simulink library "Tire_MFSwift"  (R2026a)
settings: Solver=VariableStepAuto
undefined symbols (not defined in the file): Left, UNLOADED_RADIUS, Vehicle, VERTICAL_DAMPING, VERTICAL_STIFFNESS, Visual, X, Y, Z
libraries: nesl_utility x24, sm_lib x15, mfswift_simscape_library x2, Delft_Tyre_dtlib x1, TireBody_Systems x1, mfswift_library x1, Tire_Utilities x1, $bdroot x1
(part 1 of 2)
Description:
  | Component of Simscape Vehicle Templates Library
  | 
  | Copyright 2018-2026 The MathWorks, Inc.
settings Model: Creator=smiller  LastModifiedBy=smiller

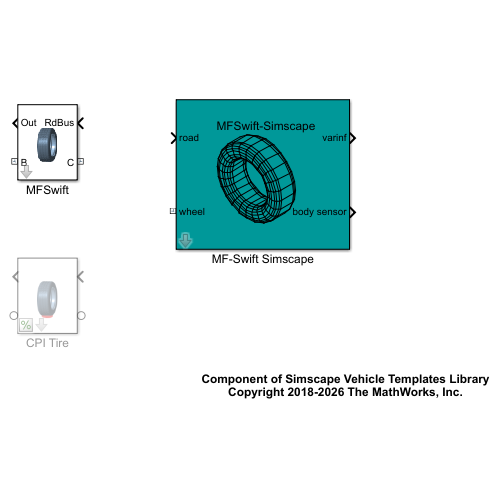
[thumbnail: Simulink's stored preview of the top-level diagram]
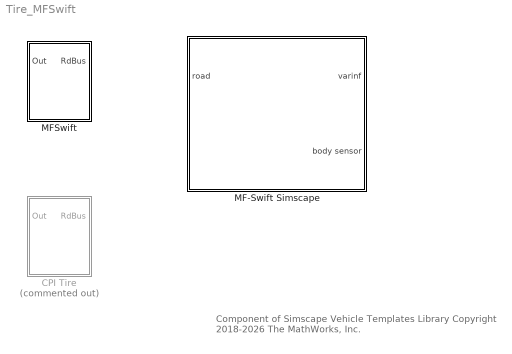
== system Tire_MFSwift ==
  note: Component of Simscape Vehicle Templates Library
      | Copyright 2018-2026 The MathWorks, Inc.
  CPI Tire : Subsystem  Commented=on  VariantControl=CPI  mask{idtyre=0}
      mask prompts: idtyre "Tyre ID [integer]"
      mask Display: image('sm_car_vehicle_tire_delftcpi_IMAGE.png');
  MF-Swift Simscape : Subsystem  Tag=STI tyre  mask(MF-Tyre/MF-Swift Simscape tire){idtyre=1, inertia=[10 1 2], tpfname=which('car213_40R21.tir'), rdfname='', road_mode=(1xxxx) default flat, side_mode=(x1xxx) left, cnt_mode=(xx1xx) smooth road, dyn_mode=(xxx2x) relaxation behaviour - non-linear, mf_mode=(xxxx4) combined, overwrite=off, use_mode=1e8, tv_model=Disabled, internal_solver=off, disp_debug=off, popup_leftRight=Left}
      mask prompts: idtyre "Tyre ID [integer]"; inertia "Rim inertia [3x real] mass(kg) Ixx Iyy (kgm2)"; tpfname "Tire properties file [string] or Tire struct [data structure]"; rdfname "Road data file [string]"; road_mode "Road method          :"; side_mode "Tyre side                :"; cnt_mode "Contact method       :"; dyn_mode "Dynamics               :"; mf_mode "Slip forces              :"; overwrite "Overwrite use mode with:"; tv_model "T&&V model               :"; internal_solver "Activate internal RK4 solver"; disp_debug "Display debug messages"; popup_leftRight "Left/Right"
      mask help:
      | MF-Tyre/MF-Swift tire model. Inputs to the tire are the motions at the wheel centre. The force and torque outputs correspond to the forces at the wheel center.
      |
      | Tire model version: MF-Tyre/MF-Swift v2021.1
      | © 2021 Siemens Industry Software and Services B.V.
      mask init:
      | curblk = gcb;
      | 
      | %radius     = 1;
      | %width      = 1;
      | %belt_mass  = 1;
      | %belt_Ixx   = 1;
      | %belt_Iyy   = 1;
      | %tyre_mass  = 1;
      | %tyre_Ixx   = 1;
      | %tyre_Iyy   = 1;
      | %mass = 1;
      | %wheelbody  = [10 1 2];
      | %Imat = [1 0 0; 0 1 0; 0 0 1];
      | 
      | idroad=1;
      | if(idtyre >= 10000 || idtyre <= 0)
      |     error('Invalid tire ID. Valid range is: 1-9999')
      | end
      | if(0 == strcmp(bdroot, 'mfswift_simscape_library'))
      |     solver_type = get_param(bdroot,'Solver');
      |     if (internal_solver)
      |         idtyre = idtyre + 10000;
      |         if(0 == strcmp(solver_type, 'ode1') && (disp_debug))
      |             warning(['ode1 solver should be used when using internal RK4 solver for more stable results'])
      |         end
      |     else
      |         if (0 == strcmp(solver_type, 'ode4')&& (disp_debug))
      |             % Disabled warning
      |             %warning(['It is recommended to use ode4 solver with external solver for more stable results'])
      |         end
      |     end
      | end
      | 
      | if strcmp(get_param(gcb,'overwrite'),'off')
      |     if cnt_mode == 3
      |         contact = 5;
      |     elseif cnt_mode == 2
      |         contact = 3;
      |     else
      |         contact = 1;
      |     end
      |     
      |     iswtch = 10000*road_mode + 1000*side_mode + 100*contact + 10*(dyn_mode-1) + (mf_mode-1);
      |     
      |     if (disp_debug) disp(['Delft-Tyre ' num2str(idtyre) ' -> use_mode=' num2str(iswtch) ]); end
      | else
      |     iswtch=use_mode;
      | end
      | 
      | currentFolder = dir;
      | hasTir = any(strcmp(tpfname, {currentFolder(~[currentFolder.isdir]).name}));
      | 
      | override_tv_mode = -1;
      | if(tv_model == 4)
      |     override_tv_mode = 3;
      | elseif(tv_model == 3)
      |     override_tv_mode = 2;
      | elseif (tv_model == 2)
      |     override_tv_mode = 1;
      | else
      |     override_tv_mode = 0;
      | end
      | 
      | typarr_updated = 0;
      | if (isstruct(tpfname))
      |     if(isfield(tpfname.MODEL, 'FITTYP'))
      |         if(tv_mode_override > 0)
      |             if(tpfname.MODEL.FITTYP < 70)
      |                 warning('For FITTYP less than 70, the T&V model is not available. The selected T&V mode will be ignored');
      |             else
      |                 tpfname.MODEL.TV_MODEL = tv_mode_override;
      |             end
      |         end
      |     end
      |     typarr = m_mfswift_struct2array(tpfname);
      |     typarr_updated = 1;
      | elseif (length(tpfname) == 0)
      |     %continue
      | elseif (hasTir == 1)
      |     typarr = m_mfswift_tirparser(tpfname, 'TV_MODE', override_tv_mode);
      |     typarr_updated = 1;
      | elseif (ischar(tpfname) && strcmp('', which(tpfname)) == 0)
      |     typarr = m_mfswift_tirparser(which(tpfname), 'TV_MODE', override_tv_mode);
      |     typarr_updated = 1;
      | else
      |     warning(['Mask parameter ''Tire property file'' should be supplied as string for tire ' num2str(idtyre)])
      |     if(length(tpfname) ~= 0)
      |         warning(['Make sure that " ' tpfname ' " is named correctly and it is available on the Matlab path or exists in the current working directory.'])
      |     end
      | end
      | 
      | tyreSimulationMode = get_param(bdroot, 'SimulationMode');
      | tyreTargetFile = get_param(bdroot, 'SystemTargetFile');
      | serialization = mfs_global_setting('serialization');
      | force_entitlement = getenv('MFSWIFTRT_FORCE_ENTITLEMENT');
      | 
      | if strcmp(force_entitlement, '1')
      |     tyreTemplateMakefile = 'force_serialization';
      | elseif strcmp(serialization, 'true')
      |     tyreTemplateMakefile = 'force_serialization';
      | else
      |     tyreTemplateMakefile = get_param(bdroot, 'TemplateMakefile');
      | end
      | 
      | % calculate the mass of the wheelbody in the MBS environment
      | %   normally           : rim + tyre
      | %   rigid ring dynamics: rim + part of tyre (and separate rigid body inside tyre model)
      | dynmod = iswtch - 100*floor(iswtch / 100);
      | dynmod = floor(dynmod / 10);
      | if (length(tpfname) == 0)
      |     %continue
      | else
      |     wheelbody = m_mfswift_wheel_property('tire_properties', tpfname, 'rim_properties', inertia, 'dynamics_mode', dynmod);
      | end
      | 
      | wheelbody_mass = wheelbody(1);
      | wheelbody_Ixx  = wheelbody(2);
      | wheelbody_Iyy  = wheelbody(3);
      | 
      | % display the use_mode of the model
      | if (disp_debug) disp(['MF-Tyre/MF-Swift ' num2str(idtyre) ' -> use_mode= ' num2str(iswtch) ]); end
      |     
      | % check and calculate inertia of the rim_body
      | %if  (inertia(1) <= 0 | inertia(2) <= 0 | inertia(3) <= 0 | wheelbody_mass <= 0 | wheelbody_Ixx <= 0 | wheelbody_Iyy <= 0 )
      | if  (wheelbody_mass <= 0 | wheelbody_Ixx <= 0 | wheelbody_Iyy <= 0 )
      |      error('Initialisation calculation results in a negative mass and/or inertia!')
      |      disp_debug=1;
      | end
      |     
      | if (disp_debug)
      |     msg=['Wheel mass = ',wheelbody_mass,' kg'];
      |     disp(msg);
      |     msg=['Wheel Ixx  = ',wheelbody_Ixx,' kgm2'];
      |     disp(msg);
      |     msg=['Wheel Iyy  = ',wheelbody_Iyy,' kgm2'];
      |     disp(msg);
      | end
      | 
      | %mass = wheelbody_mass;
      | tyre_mass = wheelbody_mass;
      | tyre_Ixx  = wheelbody_Ixx;
      | tyre_Iyy  = wheelbody_Iyy;
      | 
      | %Imat = [wheelbody_Ixx 0 0; 0 wheelbody_Iyy 0; 0 0 wheelbody_Ixx];
      | 
      | %initialize road file as uint8 with terminator character.
      | roadfile=uint8([rdfname 0]);
      | 
      | fliplr = 0;
      | % CHANGE GEOMETRY ORIENTATION IF WHEEL IS ON RIGHT SIDE
      | if (side_mode == 2)
      |     fliplr = 1;
      |     %disp(['Tyre ID = ' num2str(idtyre) ', fliplr = ' num2str(fliplr)]);
      | end
      | 
      | % Parameters needed for generic tire geometry
      | tirparams   = mfeval.readTIR(tpfname);
      | tire_radius = tirparams.UNLOADED_RADIUS;
      | tire_width  = tirparams.WIDTH;
      | rim_width   = tire_width*0.1;
      | rim_radius  = tirparams.RIM_RADIUS;
      mask Help: eval('mfs_open_help()')
      mask TypeOptions road_mode: (1xxxx) default flat | (2xxxx) opencrg | (3xxxx) external
      mask Callback road_mode:
      | enables = get_param(gcb, 'MaskEnables');
      | road = get_param(gcb,'road_mode');
      | if(road(2) == '2')
      |     enables{4} = 'on';
      | else
      |     enables{4} = 'off';
      | end
      | set_param(gcb, 'MaskEnables', enables);
      mask TypeOptions side_mode: (x1xxx) left | (x2xxx) right | (x3xxx) symmetric | (x4xxx) mirror
      mask TypeOptions cnt_mode: (xx1xx) smooth road | (xx3xx) moving road | (xx5xx) enveloping
      mask TypeOptions dyn_mode: (xxx0x) steady-state | (xxx1x) relaxation behaviour | (xxx2x) relaxation behaviour - non-linear | (xxx3x) rigid-ring
      mask TypeOptions mf_mode: (xxxx0) none | (xxxx1) longitudinal | (xxxx2) lateral | (xxxx3) uncombined | (xxxx4) combined | (xxxx5) combined+turnslip
      mask Callback overwrite:
      | enables = get_param(gcb, 'MaskEnables');
      | if strcmp(get_param(gcb,'overwrite'),'on')
      |     enables{4} = 'on';
      | 
      |     enables{5} = 'off';
      |     enables{6} = 'off';
      |     enables{7} = 'off';
      |     enables{8} = 'off';
      |     enables{9} = 'off';
      | 
      |     enables{11} = 'on';
      | else
      |     road = get_param(gcb,'road_mode');
      |     if(road(2) == '2')
      |         enables{4} = 'on';
      |     else
      |         enables{4} = 'off';
      |     end
      | 
      |     enables{5} = 'on';
      |     enables{6} = 'on';
      |     enables{7} = 'on';
      |     enables{8} = 'on';
      |     enables{9} = 'on';
      | 
      |     enables{11} = 'off';
      | end
      | set_param(gcb, 'MaskEnables', enables);
      mask TypeOptions tv_model: Disabled | Static | Dynamic without IP | Dynamic with IP
      mask TypeOptions popup_leftRight: Tire Body/popup_leftRight
      mask DialogControl cont_vis Prompt: Visualization
      mask Display:
      | text(0.3*115,0.7*178,'  MFSwift-Simscape')
      | plot(89.*[0.8828 0.8769 0.8597 0.7299 0.7043 0.6745 0.6443 0.6195 0.5884 0.5712 0.5653 0.5573 0.5346 0.4985 0.4515 0.3965 0.3373 ]+160/2-0.43*89,89.*[0.3654 0.3482 0.3335 0.2583 0.2486 0.2453 0.2486 0.2583 0.2764 0.2911 0.3083 0.2449 0.1945 0.1609 0.1462 0.1520 0.1768 ]+0.3*89)
      | plot(89.*[0.3255 0.3889 0.3965 0.4112 0.4313 0.3767 ]+160/2-0.43*89,89.*[0.1491 0.1222 0.1520 0.1777 0.1949 0.2184 ]+0.3*89)
      | plot(89.*[0.3553 0.4112 0.4633 0.4826 0.5464 ]+160/2-0.43*89,89.*[0.2012 0.1777 0.1722 0.1898 0.2268 ]+0.3*89)
      | plot(89.*[0.5426 0.5262 0.4826 0.4313 0.5603 0.5603 0.5065 ]+160/2-0.43*89,89.*[0.2184 0.2037 0.1898 0.1949 0.2692 0.2701 0.2932 ]+0.3*89)
      | plot(89.*[0.5279 0.5460 0.4868 ]+160/2-0.43*89,89.*[0.3007 0.2969 0.3402 ]+0.3*89)
      | plot(89.*[0.5279 0.5624 ]+160/2-0.43*89,89.*[0.3007 0.2856 ]+0.3*89)
      | plot(89.*[0.5628 0.5460 ]+160/2-0.43*89,89.*[0.2898 0.2969 ]+0.3*89)
      | plot(89.*[0.5712 0.5628 0.5573 ]+160/2-0.43*89,89.*[0.2911 0.2222 0.2449 ]+0.3*89)
      | plot(89.*[0.5586 0.5422 0.5082 0.4633 0.4515 0.4481 0.3889 0.3902 0.4544 0.5099 0.5523 0.5792 0.5884 ]+160/2-0.43*89,89.*[0.2541 0.2180 0.1861 0.1722 0.1462 0.1163 0.1222 0.0928 0.0865 0.1033 0.1428 0.2016 0.2764 ]+0.3*89)
      | plot(89.*[0.6195 0.6090 0.5792 0.5628 0.5380 0.5346 0.5422 ]+160/2-0.43*89,89.*[0.2583 0.1751 0.2016 0.2222 0.1680 0.1945 0.2180 ]+0.3*89)
      | plot(89.*[0.5262 0.5082 0.4985 0.4994 0.5380 0.5523 0.5792 0.6090 0.6333 0.6443 ]+160/2-0.43*89,89.*[0.2037 0.1861 0.1609 0.1319 0.1680 0.1428 0.1092 0.1751 0.1596 0.2486 ]+0.3*89)
      | plot(89.*[0.6745 0.6627 0.6333 0.6018 0.5792 0.5317 0.5099 0.4994 0.4481 0.4544 0.4700 0.5317 0.5510 0.6018 0.6291 0.6627 0.6926 0.7043 ]+160/2-0.43*89,89.*[0.2453 0.1508 0.1596 0.0890 0.1092 0.0655 0.1033 0.1319 0.1163 0.0865 0.0462 0.0655 0.0416 0.0890 0.0764 0.1508 0.1508 0.2486 ]+0.3*89)
      | plot(89.*[0.7299 0.7178 0.6926 0.6577 0.6291 0.5758 0.5510 0.4851 0.4700 0.3986 0.3213 0.2440 0.1718 0.1100 0.0626 ]+160/2-0.43*89,89.*[0.2583 0.1596 0.1508 0.0739 0.0764 0.0269 0.0416 0.0210 0.0462 0.0533 0.0861 0.1424 0.2184 0.3087 0.4074 ]+0.3*89)
      | plot(89.*[0.0487 0.0995 0.1100 0.1323 0.1516 0.1760 0.1399 ]+160/2-0.43*89,89.*[0.4082 0.3028 0.3087 0.3213 0.3326 0.3469 0.4221 ]+0.3*89)
      | plot(89.*[0.1126 0.1516 0.2024 0.2234 0.2474 0.2709 0.4011 0.4200 0.4322 0.3847 0.3486 0.3255 ]+160/2-0.43*89,89.*[0.4141 0.3326 0.2579 0.2776 0.2969 0.3121 0.3872 0.3965 0.3982 0.4670 0.5426 0.6191 ]+0.3*89)
      | plot(89.*[0.3486 0.3410 0.3755 0.3847 ]+160/2-0.43*89,89.*[0.5426 0.5330 0.4616 0.4670 ]+0.3*89)
      | plot(89.*[0.3755 0.3570 0.3234 ]+160/2-0.43*89,89.*[0.4616 0.4511 0.5212 ]+0.3*89)
      | plot(89.*[0.3570 0.2272 0.1936 ]+160/2-0.43*89,89.*[0.4511 0.3759 0.4460 ]+0.3*89)
      | plot(89.*[0.1684 0.2029 0.2272 0.2709 0.3217 0.4519 0.4721 0.4868 0.4322 ]+160/2-0.43*89,89.*[0.4334 0.3625 0.3759 0.3121 0.2583 0.3331 0.3415 0.3402 0.3982 ]+0.3*89)
      | plot(89.*[0.4200 0.3755 ]+160/2-0.43*89,89.*[0.3965 0.4616 ]+0.3*89)
      | plot(89.*[0.3570 0.4011 0.4519 0.5065 0.5279 0.4721 0.4200 ]+160/2-0.43*89,89.*[0.4511 0.3872 0.3331 0.2932 0.3007 0.3415 0.3965 ]+0.3*89)
      | plot(89.*[0.5065 0.3767 0.3217 0.2995 0.2474 0.2029 0.1760 0.2234 0.2785 0.2995 0.3553 0.3767 ]+160/2-0.43*89,89.*[0.2932 0.2184 0.2583 0.2419 0.2969 0.3625 0.3469 0.2776 0.2197 0.2419 0.2012 0.2184 ]+0.3*89)
      | plot(89.*[0.3553 0.3373 0.2785 0.2617 0.2024 0.1873 0.1323 0.0899 0.0630 0.0542 0.0231 0.0059 0.0000 0.0113 0.0168 0.0332 0.0630 0.0878 0.1172 0.1470 0.1722 0.3024 0.3192 0.3255 0.3179 0.3121 0.2948 0.1651 0.1394 0.1470 0.1172 0.0878 0.0630 0.0332 0.0168 0.0113 0.0000 ]+160/2-0.43*89,89.*[0.2012 0.1768 0.2197 0.1957 0.2579 0.2402 0.3213 0.4099 0.4994 0.5846 0.6027 0.6174 0.6346 0.5271 0.5157 0.5078 0.4994 0.4964 0.4990 0.5061 0.5174 0.5922 0.6056 0.6191 0.6917 0.6745 0.6598 0.5846 0.5745 0.6350 0.6350 0.6434 0.6594 0.6858 0.7064 0.7291 0.6346 ]+0.3*89)
      | plot(89.*[0.0059 0.0168 ]+160/2-0.43*89,89.*[0.6174 0.7064 ]+0.3*89)
      | plot(89.*[0.0113 0.0454 0.0529 0.0181 0.0113 ]+160/2-0.43*89,89.*[0.7291 0.8034 0.8270 0.7497 0.7291 ]+0.3*89)
      | plot(89.*[0.0168 0.0487 0.0454 ]+160/2-0.43*89,89.*[0.7064 0.7770 0.8034 ]+0.3*89)
      | plot(89.*[0.0487 0.0626 0.0899 0.0630 0.0542 0.0794 0.0878 0.1126 0.0899 ]+160/2-0.43*89,89.*[0.7770 0.7518 0.7182 0.6594 0.5846 0.5745 0.6434 0.6976 0.7182 ]+0.3*89)
      | plot(89.*[0.1126 0.1399 0.1684 0.1936 0.2570 ]+160/2-0.43*89,89.*[0.6976 0.6854 0.6829 0.6905 0.7274 ]+0.3*89)
      | plot(89.*[0.3011 0.1722 0.1936 ]+160/2-0.43*89,89.*[0.7182 0.6438 0.6905 ]+0.3*89)
      | plot(89.*[0.1684 0.1470 0.1722 0.1651 0.1722 0.1936 0.3234 0.3410 0.3192 0.3121 0.3163 ]+160/2-0.43*89,89.*[0.6829 0.6350 0.6438 0.5846 0.5174 0.4460 0.5212 0.5330 0.6056 0.6745 0.7119 ]+0.3*89)
      | plot(89.*[0.3200 0.3179 ]+160/2-0.43*89,89.*[0.7102 0.6917 ]+0.3*89)
      | plot(89.*[0.3020 0.2948 0.3024 0.3234 ]+160/2-0.43*89,89.*[0.7178 0.6598 0.5922 0.5212 ]+0.3*89)
      | plot(89.*[0.1470 0.1394 0.1096 0.1172 0.1399 0.1760 0.1516 0.1323 0.1100 0.0995 0.0987 0.1688 0.1806 0.1999 0.3297 0.2566 0.1264 0.0701 0.0529 0.1084 0.1264 0.1999 ]+160/2-0.43*89,89.*[0.5061 0.5745 0.5716 0.6350 0.6854 0.7190 0.7341 0.7577 0.7959 0.8240 0.8530 0.8748 0.9005 0.9185 0.9933 0.9706 0.8958 0.8438 0.8270 0.8782 0.8958 0.9185 ]+0.3*89)
      | plot(89.*[0.1806 0.1084 0.0987 0.0454 ]+160/2-0.43*89,89.*[0.9005 0.8782 0.8530 0.8034 ]+0.3*89)
      | plot(89.*[0.0487 0.0995 0.1655 0.1688 ]+160/2-0.43*89,89.*[0.7770 0.8240 0.8446 0.8748 ]+0.3*89)
      | plot(89.*[0.1655 0.1718 0.1873 0.2024 0.2234 0.2474 0.2029 0.1760 0.2234 ]+160/2-0.43*89,89.*[0.8446 0.8148 0.7745 0.7497 0.7333 0.7283 0.7144 0.7190 0.7333 ]+0.3*89)
      | plot(89.*[0.2272 0.2478 ]+160/2-0.43*89,89.*[0.7215 0.7278 ]+0.3*89)
      | plot(89.*[0.2272 0.2029 0.1684 ]+160/2-0.43*89,89.*[0.7215 0.7144 0.6829 ]+0.3*89)
      | plot(89.*[0.1936 0.2272 ]+160/2-0.43*89,89.*[0.6905 0.7215 ]+0.3*89)
      | plot(89.*[0.2024 0.1516 0.1126 ]+160/2-0.43*89,89.*[0.7497 0.7341 0.6976 ]+0.3*89)
      | plot(89.*[0.0899 0.1323 0.1873 0.2520 0.2440 0.2428 0.2499 0.2650 0.2852 0.4150 0.4372 0.3528 0.3297 0.4150 0.5065 0.5279 0.5460 0.4586 0.4372 0.5279 ]+160/2-0.43*89,89.*[0.7182 0.7577 0.7745 0.7686 0.8076 0.8370 0.8669 0.8925 0.9097 0.9849 0.9920 1.0000 0.9933 0.9849 0.9458 0.9534 0.9500 0.9870 0.9920 0.9534 ]+0.3*89)
      | plot(89.*[0.5065 0.3767 0.2852 0.1999 ]+160/2-0.43*89,89.*[0.9458 0.8711 0.9097 0.9185 ]+0.3*89)
      | plot(89.*[0.1806 0.2650 0.3553 0.3767 ]+160/2-0.43*89,89.*[0.9005 0.8925 0.8538 0.8711 ]+0.3*89)
      | plot(89.*[0.3553 0.3373 0.2499 0.1688 ]+160/2-0.43*89,89.*[0.8538 0.8295 0.8669 0.8748 ]+0.3*89)
      | plot(89.*[0.1655 0.2428 0.3255 0.3373 ]+160/2-0.43*89,89.*[0.8446 0.8370 0.8018 0.8295 ]+0.3*89)
      | plot(89.*[0.3255 0.3213 0.3213 0.3255 0.3373 0.2785 0.2617 0.3255 ]+160/2-0.43*89,89.*[0.8018 0.7749 0.7388 0.7165 0.7031 0.7278 0.7438 0.7165 ]+0.3*89)
      | plot(89.*[0.3213 0.2520 0.2617 0.2024 ]+160/2-0.43*89,89.*[0.7388 0.7686 0.7438 0.7497 ]+0.3*89)
      | plot(89.*[0.2234 0.2785 ]+160/2-0.43*89,89.*[0.7333 0.7278 ]+0.3*89)
      | plot(89.*[0.2869 0.2474 ]+160/2-0.43*89,89.*[0.7241 0.7283 ]+0.3*89)
      | plot(89.*[0.2440 0.3213 0.3986 0.4078 0.4246 0.4456 0.4683 0.5981 0.6182 0.6329 0.5460 ]+160/2-0.43*89,89.*[0.8076 0.7749 0.7186 0.7417 0.7661 0.7879 0.8043 0.8790 0.8874 0.8862 0.9500 ]+0.3*89)
      | plot(89.*[0.5279 0.6182 0.7022 0.7140 0.6329 ]+160/2-0.43*89,89.*[0.9534 0.8874 0.7984 0.8001 0.8862 ]+0.3*89)
      | plot(89.*[0.5981 0.5065 ]+160/2-0.43*89,89.*[0.8790 0.9458 ]+0.3*89)
      | plot(89.*[0.5981 0.6829 0.7022 ]+160/2-0.43*89,89.*[0.8790 0.7892 0.7984 ]+0.3*89)
      | plot(89.*[0.6829 0.5535 0.4683 0.3767 ]+160/2-0.43*89,89.*[0.7892 0.7144 0.8043 0.8711 ]+0.3*89)
      | plot(89.*[0.3553 0.4456 0.5300 0.5535 ]+160/2-0.43*89,89.*[0.8538 0.7879 0.6989 0.7144 ]+0.3*89)
      | plot(89.*[0.5300 0.5061 0.4246 0.3373 ]+160/2-0.43*89,89.*[0.6989 0.6800 0.7661 0.8295 ]+0.3*89)
      | plot(89.*[0.3255 0.4078 0.4851 0.5061 ]+160/2-0.43*89,89.*[0.8018 0.7417 0.6602 0.6800 ]+0.3*89)
      | plot(89.*[0.4851 0.4700 0.3986 0.3902 0.3889 0.4481 0.4544 0.4700 ]+160/2-0.43*89,89.*[0.6602 0.6426 0.7186 0.6884 0.6703 0.6077 0.6203 0.6426 ]+0.3*89)
      | plot(89.*[0.4851 0.5510 0.5758 0.6027 0.6262 0.7560 0.7745 0.7841 0.7140 ]+160/2-0.43*89,89.*[0.6602 0.5632 0.5779 0.5930 0.6069 0.6816 0.6926 0.6980 0.8001 ]+0.3*89)
      | plot(89.*[0.7022 0.7745 ]+160/2-0.43*89,89.*[0.7984 0.6926 ]+0.3*89)
      | plot(89.*[0.7841 0.8375 0.8303 0.7745 ]+160/2-0.43*89,89.*[0.6980 0.5863 0.5766 0.6926 ]+0.3*89)
      | plot(89.*[0.7560 0.6829 ]+160/2-0.43*89,89.*[0.6816 0.7892 ]+0.3*89)
      | plot(89.*[0.7560 0.8123 0.8303 ]+160/2-0.43*89,89.*[0.6816 0.5649 0.5766 ]+0.3*89)
      | plot(89.*[0.8123 0.6825 0.6262 0.5535 ]+160/2-0.43*89,89.*[0.5649 0.4901 0.6069 0.7144 ]+0.3*89)
      | plot(89.*[0.5300 0.6027 0.6577 0.6825 ]+160/2-0.43*89,89.*[0.6989 0.5930 0.4775 0.4901 ]+0.3*89)
      | plot(89.*[0.6577 0.6291 0.5758 0.5061 ]+160/2-0.43*89,89.*[0.4775 0.4658 0.5779 0.6800 ]+0.3*89)
      | plot(89.*[0.4700 0.5317 0.5510 0.6018 0.6291 ]+160/2-0.43*89,89.*[0.6426 0.5523 0.5632 0.4578 0.4658 ]+0.3*89)
      | plot(89.*[0.6018 0.5792 0.5317 0.5099 0.4544 0.3902 0.3213 ]+160/2-0.43*89,89.*[0.4578 0.4536 0.5523 0.5397 0.6203 0.6884 0.7388 ]+0.3*89)
      | plot(89.*[0.3255 0.3889 0.3965 0.4515 0.4481 0.4994 0.5099 0.5523 0.5792 ]+160/2-0.43*89,89.*[0.7165 0.6703 0.6602 0.6018 0.6077 0.5334 0.5397 0.4511 0.4536 ]+0.3*89)
      | plot(89.*[0.6018 0.6333 0.6627 0.6926 0.7178 0.8475 0.8652 0.8711 0.8375 ]+160/2-0.43*89,89.*[0.4578 0.3503 0.3524 0.3599 0.3713 0.4460 0.4595 0.4729 0.5863 ]+0.3*89)
      | plot(89.*[0.8303 0.8652 ]+160/2-0.43*89,89.*[0.5766 0.4595 ]+0.3*89)
      | plot(89.*[0.8711 0.8828 0.8711 0.8652 0.8475 0.7178 0.6825 0.6577 0.6027 0.5758 0.5061 0.4851 0.4078 0.3986 0.3902 0.3213 0.2520 0.1873 0.1718 0.1655 0.0995 0.0987 0.1688 0.1655 0.2428 0.2440 0.2520 0.2617 0.3255 0.3373 ]+160/2-0.43*89,89.*[0.4729 0.3654 0.2713 0.2503 0.2348 0.1596 0.0815 0.0739 0.0223 0.0269 0.0050 0.0210 0.0290 0.0533 0.0928 0.1222 0.1726 0.2402 0.2184 0.2058 0.3028 0.3020 0.1999 0.2058 0.1243 0.1424 0.1726 0.1957 0.1491 0.1768 ]+0.3*89)
      | plot(89.*[0.3255 0.3213 0.3213 0.3255 0.4078 0.4246 0.5061 0.5300 0.6027 0.6262 0.6825 0.8123 0.8475 0.8597 0.8475 0.8123 ]+160/2-0.43*89,89.*[0.1491 0.1222 0.0861 0.0643 0.0290 0.0130 0.0050 0.0000 0.0223 0.0294 0.0815 0.1562 0.2348 0.3335 0.4460 0.5649 ]+0.3*89)
      | plot(89.*[0.8652 0.8769 0.8652 0.8303 0.8123 0.7560 0.6262 0.5535 0.5300 0.4456 0.4246 0.3373 0.3255 0.2428 0.2499 0.3373 ]+160/2-0.43*89,89.*[0.4595 0.3482 0.2503 0.1735 0.1562 0.1046 0.0294 0.0067 0.0000 0.0084 0.0130 0.0504 0.0643 0.1243 0.1138 0.0504 ]+0.3*89)
      | plot(89.*[0.0487 0.0168 0.0059 ]+160/2-0.43*89,89.*[0.4082 0.5157 0.6174 ]+0.3*89)
      | plot(89.*[0.0231 0.0332 0.0626 0.1100 0.1718 0.2440 ]+160/2-0.43*89,89.*[0.6027 0.6858 0.7518 0.7959 0.8148 0.8076 ]+0.3*89)
      | plot(89.*[0.3373 0.3965 ]+160/2-0.43*89,89.*[0.7031 0.6602 ]+0.3*89)
      | plot(89.*[0.4515 0.4985 0.4994 0.5380 0.5523 0.5792 0.6090 0.6333 0.6443 ]+160/2-0.43*89,89.*[0.6018 0.5330 0.5334 0.4519 0.4511 0.3612 0.3532 0.3503 0.2486 ]+0.3*89)
      | plot(89.*[0.6745 0.6627 0.6291 ]+160/2-0.43*89,89.*[0.2453 0.3524 0.4658 ]+0.3*89)
      | plot(89.*[0.6577 0.6926 0.7043 ]+160/2-0.43*89,89.*[0.4775 0.3599 0.2486 ]+0.3*89)
      | plot(89.*[0.7299 0.7178 0.6825 ]+160/2-0.43*89,89.*[0.2583 0.3713 0.4901 ]+0.3*89)
      | plot(89.*[0.5792 0.6090 0.6195 ]+160/2-0.43*89,89.*[0.4536 0.3532 0.2583 ]+0.3*89)
      | plot(89.*[0.5884 0.5792 0.5628 0.5380 0.5346 0.5573 0.5628 0.5712 ]+160/2-0.43*89,89.*[0.2764 0.3612 0.3692 0.4519 0.4578 0.3809 0.3692 0.2911 ]+0.3*89)
      | plot(89.*[0.5653 0.5573 ]+160/2-0.43*89,89.*[0.3083 0.3809 ]+0.3*89)
      | plot(89.*[0.5346 0.4985 ]+160/2-0.43*89,89.*[0.4578 0.5330 ]+0.3*89)
      | plot(89.*[0.1470 0.1684 0.1936 ]+160/2-0.43*89,89.*[0.5061 0.4334 0.4460 ]+0.3*89)
      | plot(89.*[0.1684 0.1399 0.1172 0.1096 0.0794 0.0878 0.1126 0.1399 ]+160/2-0.43*89,89.*[0.4334 0.4221 0.4990 0.5716 0.5745 0.4964 0.4141 0.4221 ]+0.3*89)
      | plot(89.*[0.1126 0.0899 0.0626 0.0332 0.0231 ]+160/2-0.43*89,89.*[0.4141 0.4099 0.4074 0.5078 0.6027 ]+0.3*89)
      | plot(89.*[0.0113 0.0454 0.0487 0.0626 ]+160/2-0.43*89,89.*[0.5271 0.4137 0.4082 0.4074 ]+0.3*89)
      | plot(89.*[0.0454 0.0987 ]+160/2-0.43*89,89.*[0.4137 0.3020 ]+0.3*89)
  MFSwift : Subsystem  VariantControl=Delft  mask(MF-Swift Tire){idtyre=2, rim_inertia=Vehicle.Chassis.TireA1.mjRim.Value, tir_name=Vehicle.Chassis.TireA1.tirFile.Value, rdf_name=Vehicle.Chassis.TireA1.roadFile.Value, tire_side_mode=(x2xxx) right, tire_contact=Vehicle.Chassis.TireA1.Contact.Value, tire_dynamics=Vehicle.Chassis.TireA1.Dynamics.Value, tire_slip=Vehicle.Chassis.TireA1.Slip.Value, solver_enable=Vehicle.Chassis.TireA1.InternalSolver.Value, TireBody=Vehicle.Chassis.TireA1.TireBody, popup_leftRight=Right, clr_tyre=Visual.Tire.clr, opc_tyre=Visual.Tire.opc, clr_rim=Visual.Rim.clr, opc_rim=Visual.Rim.opc}
      mask prompts: idtyre "Tyre ID [integer]"; rim_inertia "Rim: [Mass (kg) Ixx Iyy (kg*m2)]"; tir_name "Tyre properties [string or struct]"; rdf_name "Road data file [string]"; tire_side_mode "Tyre Side"; tire_contact "Contact Method"; tire_dynamics "Dynamics Mode"; tire_slip "Slip Mode"; solver_enable "Enable Internal Solver"; TireBody "Tire Body (structure)"; popup_leftRight "Left/Right"
      mask init:
      | curblk = gcb;
      | 
      | set_param([gcb '/Wheel and Tyre'],'cnt_mode',tire_contact);
      | set_param([gcb '/Wheel and Tyre'],'dyn_mode',tire_dynamics);
      | set_param([gcb '/Wheel and Tyre'],'mf_mode',tire_slip);
      | set_param([gcb '/Wheel and Tyre'],'tpfname',tir_name);
      | set_param([gcb '/Wheel and Tyre'],'rdfname',rdf_name);
      | 
      | % Set road_mode parameter based on road file type
      | if(contains(lower(rdf_name),'.crg'))
      |     set_param([gcb,'/Wheel and Tyre'],'road_mode','(2xxxx) opencrg');
      |     set_param([gcb,'/Road Inputs'],'LabelModeActiveChoice','NonMoving');
      | else
      |     set_param([gcb '/Wheel and Tyre'],'rdfname','''''');
      |     if(contains(lower(rdf_name),'external'))
      |         set_param([gcb,'/Wheel and Tyre'],'road_mode','(3xxxx) external');
      |         set_param([gcb,'/Road Inputs'],'LabelModeActiveChoice','ExternalRoad');
      |     else
      |         set_param([gcb,'/Wheel and Tyre'],'road_mode','(1xxxx) default flat');
      |         set_param([gcb,'/Road Inputs'],'LabelModeActiveChoice','NonMoving');
      |     end
      | end
      | 
      | % Enable or disable internal solver
      | if(strcmp(lower(solver_enable),'on'))
      |     set_param([gcb '/Wheel and Tyre'],'internal_solver','on');
      | else
      |     set_param([gcb '/Wheel and Tyre'],'internal_solver','off');
      | end
      |    
      | if(popup_leftRight == 1)
      |     set_param([gcb '/Wheel and Tyre'],'popup_leftRight','Left');
      | elseif(popup_leftRight == 2)
      |     set_param([gcb '/Wheel and Tyre'],'popup_leftRight','Right');
      | end
      mask TypeOptions idtyre: Wheel and Tyre/idtyre
      mask TypeOptions rim_inertia: Wheel and Tyre/inertia
      mask TypeOptions tire_side_mode: Wheel and Tyre/side_mode
      mask TypeOptions popup_leftRight: Left | Right
      mask TypeOptions clr_tyre: Wheel and Tyre/clr_tyre
      mask TypeOptions opc_tyre: Wheel and Tyre/opc_tyre
      mask TypeOptions clr_rim: Wheel and Tyre/clr_rim
      mask TypeOptions opc_rim: Wheel and Tyre/opc_rim
      mask DialogControl cont_tire_delft Prompt: Tire
      mask DialogControl cont_vis Prompt: Visualization
      mask DialogControl text_tire_clr Prompt: Color [RGB]
      mask DialogControl text_tire_opc Prompt: Opacity (0-1)
      mask DialogControl text_tire Prompt: Tyre
      mask DialogControl text_rim Prompt: Rim
      mask Display: image('sm_car_vehicle_tire_delft_IMAGE.png');

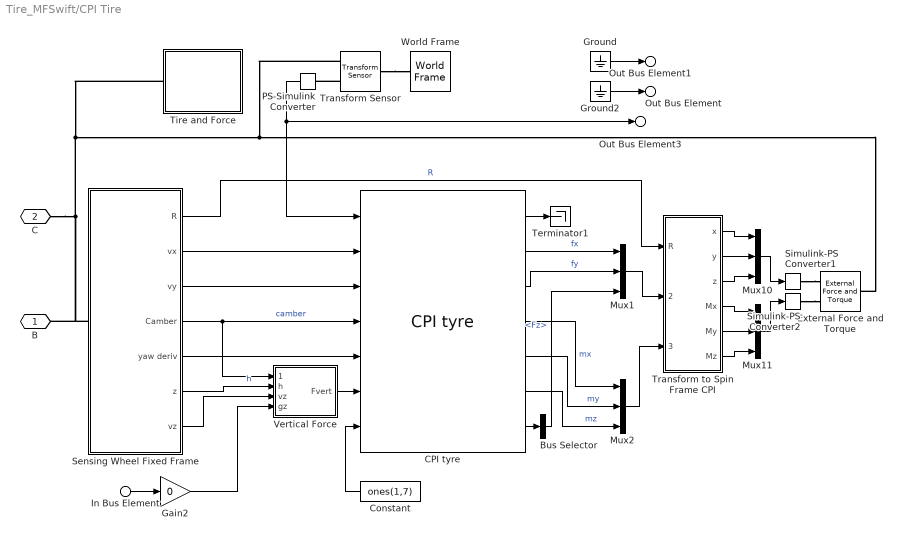
== system Tire_MFSwift/CPI Tire ==
  In Bus Element : Inport  PortName=RdBus  Element=RdBus
  Bus Selector : BusSelector  OutputSignals=Fz
  CPI tyre : Delft_Tyre_dtlib/Simulink/CPI tyre  Tag=CPI tyre  idtyre=1  tpfname=[]  side_mode=(1xxx) left  dyn_mode=(xx0x) steady-state  mf_mode=(xxx0) none  use_mode=1e8  disp_debug=off
  Constant : Constant  Value=ones(1,7)
  External Force and Torque : sm_lib/Forces and Torques/External Force and Torque  EnableForceX=off  EnableForceY=off  EnableForceZ=off  EnableForce=on  ForceResolutionFrame=AttachedFrame  EnableTorqueX=off  EnableTorqueY=off  EnableTorqueZ=off  EnableTorque=on  TorqueResolutionFrame=AttachedFrame
  Gain2 : Gain  Gain=0
  Ground : Ground
  Ground2 : Ground
  Mux{1..2,10..11} (4 alike) : Mux  Inputs=3
  PS-Simulink Converter : nesl_utility/PS-Simulink Converter  PhysicalDomain=network_engine_domain  SubClassName=ps_output  LeftPortType=input  RightPortType=output  PseudoPeriodic=off  Frequencies=[]  VectorFormat=1-D array  Unit=1  AffineConversion=off
  Sensing Wheel Fixed Frame : Subsystem
  Simulink-PS Converter1 : nesl_utility/Simulink-PS Converter  PhysicalDomain=network_engine_domain  SubClassName=ps_input  LeftPortType=input  RightPortType=output  PseudoPeriodic=off  Frequencies=[]  NoiseDistribution=none  NoiseParameters=[]  Unit=N  AffineConversion=off  FilteringAndDerivatives=provide  SimscapeFilterOrder=1  InputFilterTimeConstant=0.001  UdotUserProvided=0
  Simulink-PS Converter2 : nesl_utility/Simulink-PS Converter  PhysicalDomain=network_engine_domain  SubClassName=ps_input  LeftPortType=input  RightPortType=output  PseudoPeriodic=off  Frequencies=[]  NoiseDistribution=none  NoiseParameters=[]  Unit=N*m  AffineConversion=off  FilteringAndDerivatives=provide  SimscapeFilterOrder=1  InputFilterTimeConstant=0.001  UdotUserProvided=0
  Terminator1 : Terminator
  Tire and Force : Subsystem  mask{radius=0.4225, rim_radius=0.3048, width=0.235, rim_width=0.235*0.1, mass=10, rim_mass=0, tire_inertia=[1 2], rim_inertia=[0 0], clr_tyre_cfl=[0.5 0.5 0.5], opc_tyre_cfl=1.0, clr_rim_cfl=[0.8 0.8 0.8], opc_rim_cfl=0.5}
      mask init:
      | Imat = [tire_inertia(1)+rim_inertia(1) 0 0; 0 tire_inertia(2)+rim_inertia(2) 0; 0 0 tire_inertia(1)+rim_inertia(1)];
      mask TypeOptions clr_tyre_cfl: Tire/GraphicDiffuseColor
      mask TypeOptions opc_tyre_cfl: Tire/GraphicOpacity
      mask TypeOptions clr_rim_cfl: Rim/GraphicDiffuseColor
      mask TypeOptions opc_rim_cfl: Rim/GraphicOpacity
      mask DialogControl cont_tyre_cfl Prompt: Contact Force Tyre
      mask DialogControl group_tyre_dim Prompt: Dimensions
      mask DialogControl text_tyre_tire Prompt: Tyre
      mask DialogControl text_tyre_rim Prompt: Rim
      mask DialogControl text_tyre_dim_radius Prompt: Radius (m)
      mask DialogControl text_tyre_dim_width Prompt: Width (m)
      mask DialogControl text_tyre_mass Prompt: Mass (kg)
      mask DialogControl text_tyre_inertia Prompt: Inertia [Ixx Iyy]
      mask DialogControl cont_tyre_cfl_vis Prompt: Visualization
      mask DialogControl text_vis_tyre_cfl_clr Prompt: Color [RGB]
      mask DialogControl text_vis_tyre_cfl_opc Prompt: Opacity (0-1)
      mask DialogControl text_vis_tyre_tyre Prompt: Tyre
      mask DialogControl text_vis_tyre_rim Prompt: Rim
  Transform Sensor : sm_lib/Frames and Transforms/Transform Sensor  MeasurementFrame=NonRotatingFollower  RotationSequence=XYX  SenseAngle=off  SenseAxis=off  SenseQ=off  SenseR=off  SenseRotationSequence=off  SenseOmegaX=off  SenseOmegaY=off  SenseOmegaZ=on  SenseOmega=off  SenseQDot=off  SenseRDot=off  SenseRotationSequenceDot=off  SenseAlphaX=off  SenseAlphaY=off  SenseAlphaZ=off  SenseAlpha=off  SenseQDDot=off  SenseRDDot=off  SenseX=off  SenseY=off  SenseZ=off  SenseXYZ=off  SenseRad=off  SenseAzim=off  SenseDist=off  SenseInc=off  SenseXDot=off  SenseYDot=off  SenseZDot=off  SenseXYZDot=off  SenseRadDot=off  SenseAzimDot=off  SenseDistDot=off  SenseIncDot=off  SenseXDDot=off  SenseYDDot=off  SenseZDDot=off  SenseXYZDDot=off  SenseRadDDot=off  SenseAzimDDot=off  SenseDistDDot=off  SenseIncDDot=off
  Transform to Spin Frame CPI : Subsystem
  Vertical Force : Subsystem
  World Frame : sm_lib/Frames and Transforms/World Frame
  B : PMIOPort  Side=Right
  C : PMIOPort  Port=2  Side=Left
  Out Bus Element : Outport  VectorParamsAs1DForOutWhenUnconnected=off  PortName=Out  Element=qxyz
  Out Bus Element1 : Outport  VectorParamsAs1DForOutWhenUnconnected=off  PortName=Out  Element=xyz
  Out Bus Element3 : Outport  VectorParamsAs1DForOutWhenUnconnected=off  PortName=Out  Element=omega
  wires:
  Mux1/1 -> Transform to Spin Frame CPI/2(Fcontact)
  Mux2/1 -> Transform to Spin Frame CPI/3(MContact)
  Mux10/1 -> Simulink-PS Converter1/1
  Transform to Spin Frame CPI/2(y) -> Mux10/2
  Transform to Spin Frame CPI/3(z) -> Mux10/3
  Transform to Spin Frame CPI/5(My) -> Mux11/2
  Transform to Spin Frame CPI/4(Mx) -> Mux11/1
  Transform to Spin Frame CPI/6(Mz) -> Mux11/3
  Transform to Spin Frame CPI/1(x) -> Mux10/1
  Mux11/1 -> Simulink-PS Converter2/1
  Gain2/1 -> Vertical Force/4(gz)
  Sensing Wheel Fixed Frame/7(vz) -> Vertical Force/3(vz)
  Sensing Wheel Fixed Frame/6(z) -> Vertical Force/2(h)  "h"
  Sensing Wheel Fixed Frame/4(Camber) -> Vertical Force/1(camber), CPI tyre/4  "camber"
  CPI tyre/1 -> Terminator1/1
  PS-Simulink Converter/1 -> Out Bus Element3/1, CPI tyre/1
  Sensing Wheel Fixed Frame/2(vx) -> CPI tyre/2
  CPI tyre/4 -> Mux2/1  "mx"
  CPI tyre/3 -> Mux1/2  "fy"
  Constant/1 -> CPI tyre/7
  CPI tyre/5 -> Mux2/2  "my"
  CPI tyre/6 -> Mux2/3  "mz"
  Bus Selector/1 -> Mux1/3  "<Fz>"
  CPI tyre/2 -> Mux1/1  "fx"
  Vertical Force/1(Fvert) -> CPI tyre/6
  Sensing Wheel Fixed Frame/3(vy) -> CPI tyre/3
  Sensing Wheel Fixed Frame/5(yaw deriv) -> CPI tyre/5
  Sensing Wheel Fixed Frame/1(R) -> Transform to Spin Frame CPI/1(R)  "R"
  CPI tyre/7 -> Bus Selector/1
  Ground2/1 -> Out Bus Element/1
  Ground/1 -> Out Bus Element1/1
  In Bus Element/1 -> Gain2/1
  connections:
  Simulink-PS Converter1/RConn1 -- External Force and Torque/LConn1
  Simulink-PS Converter2/RConn1 -- External Force and Torque/LConn2
  Tire and Force/LConn1 -- Sensing Wheel Fixed Frame/LConn1 -- B/RConn1 -- C/RConn1 -- Transform Sensor/RConn1 -- External Force and Torque/RConn1
  Transform Sensor/LConn1 -- World Frame/RConn1
  Transform Sensor/RConn2 -- PS-Simulink Converter/LConn1

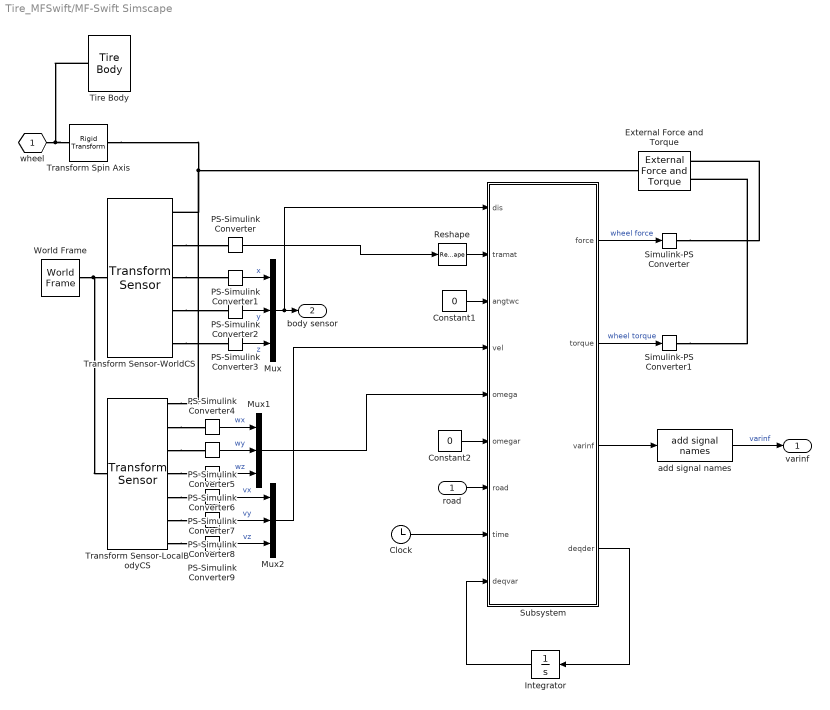
== system Tire_MFSwift/MF-Swift Simscape ==
  road : Inport
  Clock : Clock
  Constant1 : Constant  Value=0
  Constant2 : Constant  Value=0
  External Force and Torque : sm_lib/Forces and Torques/External Force and Torque  EnableForceX=off  EnableForceY=off  EnableForceZ=off  EnableForce=on  ForceResolutionFrame=AttachedFrame  EnableTorqueX=off  EnableTorqueY=off  EnableTorqueZ=off  EnableTorque=on  TorqueResolutionFrame=AttachedFrame
  Integrator : Integrator
  Mux : Mux  Inputs=3
  Mux1 : Mux  Inputs=3
  Mux2 : Mux  Inputs=3
  PS-Simulink Converter{,1..9} (10 alike) : nesl_utility/PS-Simulink Converter  PhysicalDomain=network_engine_domain  SubClassName=ps_output  LeftPortType=input  RightPortType=output  PseudoPeriodic=off  Frequencies=[]  VectorFormat=1-D array  Unit=1  AffineConversion=off
  Reshape : Reshape
  Simulink-PS Converter : nesl_utility/Simulink-PS Converter  PhysicalDomain=network_engine_domain  SubClassName=ps_input  LeftPortType=input  RightPortType=output  PseudoPeriodic=off  Frequencies=[]  NoiseDistribution=none  NoiseParameters=[]  Unit=1  AffineConversion=off  FilteringAndDerivatives=zero  SimscapeFilterOrder=1  InputFilterTimeConstant=0.001  UdotUserProvided=1
  Simulink-PS Converter1 : nesl_utility/Simulink-PS Converter  PhysicalDomain=network_engine_domain  SubClassName=ps_input  LeftPortType=input  RightPortType=output  PseudoPeriodic=off  Frequencies=[]  NoiseDistribution=none  NoiseParameters=[]  Unit=1  AffineConversion=off  FilteringAndDerivatives=zero  SimscapeFilterOrder=1  InputFilterTimeConstant=0.001  UdotUserProvided=1
  Subsystem : Subsystem
  Tire Body : TireBody_Systems/Tire Body  LabelModeActiveChoice=CAD_213_40R21  popup_leftRight=Left  TireBody=Tire.TireBody  VariantLabel=Tire.TireBody.class.Value
      settings: AttributesFormatString=%<LabelModeActiveChoice>
  Transform Sensor-LocalBodyCS : sm_lib/Frames and Transforms/Transform Sensor  MeasurementFrame=NonRotatingFollower  RotationSequence=XYX  SenseAngle=off  SenseAxis=off  SenseQ=off  SenseR=off  SenseRotationSequence=off  SenseOmegaX=on  SenseOmegaY=on  SenseOmegaZ=on  SenseOmega=off  SenseQDot=off  SenseRDot=off  SenseRotationSequenceDot=off  SenseAlphaX=off  SenseAlphaY=off  SenseAlphaZ=off  SenseAlpha=off  SenseQDDot=off  SenseRDDot=off  SenseX=off  SenseY=off  SenseZ=off  SenseXYZ=off  SenseRad=off  SenseAzim=off  SenseDist=off  SenseInc=off  SenseXDot=on  SenseYDot=on  SenseZDot=on  SenseXYZDot=off  SenseRadDot=off  SenseAzimDot=off  SenseDistDot=off  SenseIncDot=off  SenseXDDot=off  SenseYDDot=off  SenseZDDot=off  SenseXYZDDot=off  SenseRadDDot=off  SenseAzimDDot=off  SenseDistDDot=off  SenseIncDDot=off
  Transform Sensor-WorldCS : sm_lib/Frames and Transforms/Transform Sensor  MeasurementFrame=World  RotationSequence=XYX  SenseAngle=off  SenseAxis=off  SenseQ=off  SenseR=on  SenseRotationSequence=off  SenseOmegaX=off  SenseOmegaY=off  SenseOmegaZ=off  SenseOmega=off  SenseQDot=off  SenseRDot=off  SenseRotationSequenceDot=off  SenseAlphaX=off  SenseAlphaY=off  SenseAlphaZ=off  SenseAlpha=off  SenseQDDot=off  SenseRDDot=off  SenseX=on  SenseY=on  SenseZ=on  SenseXYZ=off  SenseRad=off  SenseAzim=off  SenseDist=off  SenseInc=off  SenseXDot=off  SenseYDot=off  SenseZDot=off  SenseXYZDot=off  SenseRadDot=off  SenseAzimDot=off  SenseDistDot=off  SenseIncDot=off  SenseXDDot=off  SenseYDDot=off  SenseZDDot=off  SenseXYZDDot=off  SenseRadDDot=off  SenseAzimDDot=off  SenseDistDDot=off  SenseIncDDot=off
  Transform Spin Axis : sm_lib/Frames and Transforms/Rigid Transform  RotationMethod=StandardAxis  FollAlignAxisA=+X  BaseAlignAxisA=+Y  FollAlignAxisB=+Y  BaseAlignAxisB=+Z  RotationStandardAxis=-X  RotationAngle=90  RotationAngleUnits=deg  RotationArbitraryAxis=[0 0 1]  RotationSequenceAxes=FollowerAxes  RotationSequence=XYX  RotationSequenceAngles=[0 0 0]  RotationSequenceAnglesUnits=deg  RotationMatrix=[1 0 0; 0 1 0; 0 0 1]  Quaternion=[1 0 0 0]  TranslationMethod=None  TranslationCartesianOffset=[0 0 0]  TranslationCartesianOffsetUnits=m  TranslationStandardAxis=+Z  TranslationStandardOffset=0  TranslationStandardOffsetUnits=m  TranslationROffset=0  TranslationROffsetUnits=m  TranslationThetaOffset=0  TranslationThetaOffsetUnits=deg  TranslationZOffset=0  TranslationZOffsetUnits=m
  World Frame : sm_lib/Frames and Transforms/World Frame
  add signal names : mfswift_library/MF-Swift/add signal names  SystemSampleTime=-1  VariantActivationTime=update diagram  EmptyChoice=off  PassThrough=off  PassThroughVariantControl=(default)  EmptyChoiceVariantControl=(default)  AllowFlexibleInterface=on  Latency=0  AutoFrameSizeCalculation=off
      settings: SourceProductName=MF-Tyre/MF-Swift Library
  wheel : PMIOPort  Side=Left
  varinf : Outport
  body sensor : Outport  Port=2
  wires:
  Clock/1 -> Subsystem/8(time)
  Integrator/1 -> Subsystem/9(deqvar)
  Subsystem/4(deqder) -> Integrator/1
  Subsystem/3(varinf) -> add signal names/1
  add signal names/1 -> varinf/1  "varinf"
  PS-Simulink Converter4/1 -> Mux1/1  "wx"
  PS-Simulink Converter9/1 -> Mux2/3  "vz"
  PS-Simulink Converter8/1 -> Mux2/2  "vy"
  PS-Simulink Converter7/1 -> Mux2/1  "vx"
  PS-Simulink Converter5/1 -> Mux1/2  "wy"
  Mux/1 -> Subsystem/1(dis), body sensor/1
  PS-Simulink Converter3/1 -> Mux/3  "z"
  PS-Simulink Converter2/1 -> Mux/2  "y"
  Mux2/1 -> Subsystem/4(vel)
  PS-Simulink Converter1/1 -> Mux/1  "x"
  PS-Simulink Converter6/1 -> Mux1/3  "wz"
  Mux1/1 -> Subsystem/5(omega)
  Subsystem/2(torque) -> Simulink-PS Converter1/1  "wheel torque"
  Subsystem/1(force) -> Simulink-PS Converter/1  "wheel force"
  Reshape/1 -> Subsystem/2(tramat)
  PS-Simulink Converter/1 -> Reshape/1
  Constant1/1 -> Subsystem/3(angtwc)
  road/1 -> Subsystem/7(road)
  Constant2/1 -> Subsystem/6(omegar)
  connections:
  World Frame/RConn1 -- Transform Sensor-WorldCS/LConn1 -- Transform Sensor-LocalBodyCS/LConn1
  Transform Spin Axis/LConn1 -- External Force and Torque/RConn1 -- Transform Sensor-LocalBodyCS/RConn1 -- Transform Sensor-WorldCS/RConn1
  Transform Sensor-LocalBodyCS/RConn7 -- PS-Simulink Converter9/LConn1
  Transform Sensor-WorldCS/RConn2 -- PS-Simulink Converter/LConn1
  Transform Sensor-LocalBodyCS/RConn6 -- PS-Simulink Converter8/LConn1
  Transform Sensor-WorldCS/RConn4 -- PS-Simulink Converter2/LConn1
  Transform Sensor-WorldCS/RConn3 -- PS-Simulink Converter1/LConn1
  Transform Sensor-LocalBodyCS/RConn5 -- PS-Simulink Converter7/LConn1
  Transform Sensor-WorldCS/RConn5 -- PS-Simulink Converter3/LConn1
  Transform Sensor-LocalBodyCS/RConn3 -- PS-Simulink Converter5/LConn1
  wheel/RConn1 -- Tire Body/LConn1 -- Transform Spin Axis/RConn1
  Transform Sensor-LocalBodyCS/RConn2 -- PS-Simulink Converter4/LConn1
  Transform Sensor-LocalBodyCS/RConn4 -- PS-Simulink Converter6/LConn1
  Simulink-PS Converter/RConn1 -- External Force and Torque/LConn1
  Simulink-PS Converter1/RConn1 -- External Force and Torque/LConn2

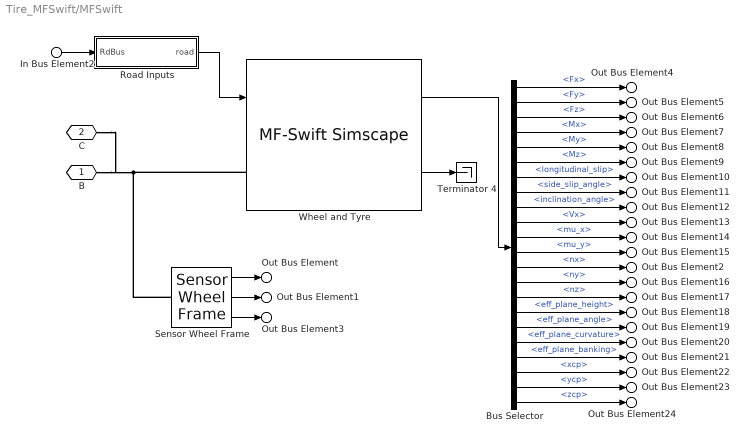
== system Tire_MFSwift/MFSwift ==
  In Bus Element2 : Inport  PortName=RdBus
  Bus Selector : BusSelector  OutputSignals=Fx,Fy,Fz,Mx,My,Mz,longitudinal_slip,side_slip_angle,inclination_angle,Vx,mu_x,mu_y,nx,ny,nz,eff_plane_height,eff_plane_angle,eff_plane_curvature,eff_plane_banking,xcp,ycp,zcp
  Road Inputs : Subsystem  Variant=on  VariantControlMode=label  LabelModeActiveChoice=ExternalRoad
  Sensor Wheel Frame : Tire_Utilities/Sensor Wheel Frame  SystemSampleTime=-1  VariantActivationTime=update diagram  EmptyChoice=off  PassThrough=off  PassThroughVariantControl=(default)  EmptyChoiceVariantControl=(default)  AllowFlexibleInterface=on  Latency=0  AutoFrameSizeCalculation=off
  Terminator 4 : Terminator
  Wheel and Tyre : $bdroot/MF-Swift Simscape  Tag=STI tyre  idtyre=idtyre  inertia=rim_inertia  tpfname=which('car213_40R21.tir')  rdfname=''  road_mode=(3xxxx) external  side_mode=(x2xxx) right  cnt_mode=(xx3xx) moving road  dyn_mode=(xxx0x) steady-state  mf_mode=(xxxx4) combined  overwrite=off  use_mode=1e8  tv_model=Disabled  internal_solver=off  disp_debug=off  popup_leftRight=Right
  B : PMIOPort  Side=Right
  C : PMIOPort  Port=2  Side=Left
  Out Bus Element : Outport  VectorParamsAs1DForOutWhenUnconnected=off  PortName=Out  Element=qxyz
  Out Bus Element1 : Outport  VectorParamsAs1DForOutWhenUnconnected=off  PortName=Out  Element=xyz
  Out Bus Element3 : Outport  VectorParamsAs1DForOutWhenUnconnected=off  PortName=Out  Element=n
  Out Bus Element4 : Outport  VectorParamsAs1DForOutWhenUnconnected=off  PortName=Out  Element=Fx
  Out Bus Element5 : Outport  VectorParamsAs1DForOutWhenUnconnected=off  PortName=Out  Element=Fy
  Out Bus Element6 : Outport  VectorParamsAs1DForOutWhenUnconnected=off  PortName=Out  Element=Fz
  Out Bus Element7 : Outport  VectorParamsAs1DForOutWhenUnconnected=off  PortName=Out  Element=Mx
  Out Bus Element8 : Outport  VectorParamsAs1DForOutWhenUnconnected=off  PortName=Out  Element=My
  Out Bus Element9 : Outport  VectorParamsAs1DForOutWhenUnconnected=off  PortName=Out  Element=Mz
  Out Bus Element10 : Outport  VectorParamsAs1DForOutWhenUnconnected=off  PortName=Out  Element=rSlip
  Out Bus Element11 : Outport  VectorParamsAs1DForOutWhenUnconnected=off  PortName=Out  Element=aSlip
  Out Bus Element12 : Outport  VectorParamsAs1DForOutWhenUnconnected=off  PortName=Out  Element=aCamber
  Out Bus Element13 : Outport  VectorParamsAs1DForOutWhenUnconnected=off  PortName=Out  Element=vx
  Out Bus Element14 : Outport  VectorParamsAs1DForOutWhenUnconnected=off  PortName=Out  Element=rMuX
  Out Bus Element15 : Outport  VectorParamsAs1DForOutWhenUnconnected=off  PortName=Out  Element=rMuY
  Out Bus Element2 : Outport  VectorParamsAs1DForOutWhenUnconnected=off  PortName=Out  Element=uvec_x
  Out Bus Element16 : Outport  VectorParamsAs1DForOutWhenUnconnected=off  PortName=Out  Element=uvec_y
  Out Bus Element17 : Outport  VectorParamsAs1DForOutWhenUnconnected=off  PortName=Out  Element=uvec_z
  Out Bus Element18 : Outport  VectorParamsAs1DForOutWhenUnconnected=off  PortName=Out  Element=pl_height
  Out Bus Element19 : Outport  VectorParamsAs1DForOutWhenUnconnected=off  PortName=Out  Element=pl_angle
  Out Bus Element20 : Outport  VectorParamsAs1DForOutWhenUnconnected=off  PortName=Out  Element=pl_curve
  Out Bus Element21 : Outport  VectorParamsAs1DForOutWhenUnconnected=off  PortName=Out  Element=pl_bank
  Out Bus Element22 : Outport  VectorParamsAs1DForOutWhenUnconnected=off  PortName=Out  Element=xcp
  Out Bus Element23 : Outport  VectorParamsAs1DForOutWhenUnconnected=off  PortName=Out  Element=ycp
  Out Bus Element24 : Outport  VectorParamsAs1DForOutWhenUnconnected=off  PortName=Out  Element=zcp
  wires:
  Bus Selector/2 -> Out Bus Element5/1  "<Fy>"
  Bus Selector/3 -> Out Bus Element6/1  "<Fz>"
  Bus Selector/10 -> Out Bus Element13/1  "<Vx>"
  Wheel and Tyre/1 -> Bus Selector/1
  Bus Selector/8 -> Out Bus Element11/1  "<side_slip_angle>"
  Bus Selector/11 -> Out Bus Element14/1  "<mu_x>"
  Bus Selector/1 -> Out Bus Element4/1  "<Fx>"
  Bus Selector/12 -> Out Bus Element15/1  "<mu_y>"
  Bus Selector/6 -> Out Bus Element9/1  "<Mz>"
  Bus Selector/7 -> Out Bus Element10/1  "<longitudinal_slip>"
  Bus Selector/9 -> Out Bus Element12/1  "<inclination_angle>"
  Bus Selector/4 -> Out Bus Element7/1  "<Mx>"
  Bus Selector/5 -> Out Bus Element8/1  "<My>"
  Sensor Wheel Frame/3 -> Out Bus Element3/1
  Sensor Wheel Frame/2 -> Out Bus Element1/1
  Sensor Wheel Frame/1 -> Out Bus Element/1
  Road Inputs/1(road) -> Wheel and Tyre/1
  Wheel and Tyre/2 -> Terminator 4/1
  In Bus Element2/1 -> Road Inputs/1(RdBus)
  Bus Selector/13 -> Out Bus Element2/1  "<nx>"
  Bus Selector/14 -> Out Bus Element16/1  "<ny>"
  Bus Selector/15 -> Out Bus Element17/1  "<nz>"
  Bus Selector/16 -> Out Bus Element18/1  "<eff_plane_height>"
  Bus Selector/17 -> Out Bus Element19/1  "<eff_plane_angle>"
  Bus Selector/18 -> Out Bus Element20/1  "<eff_plane_curvature>"
  Bus Selector/19 -> Out Bus Element21/1  "<eff_plane_banking>"
  Bus Selector/20 -> Out Bus Element22/1  "<xcp>"
  Bus Selector/21 -> Out Bus Element23/1  "<ycp>"
  Bus Selector/22 -> Out Bus Element24/1  "<zcp>"
  connections:
  Sensor Wheel Frame/LConn1 -- Wheel and Tyre/LConn1 -- B/RConn1 -- C/RConn1

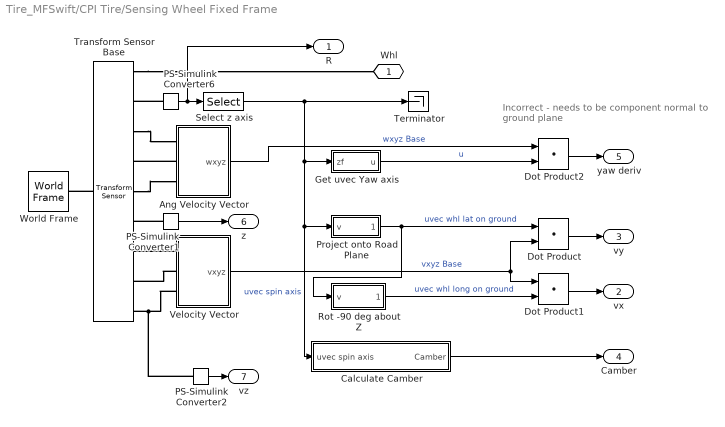
== system Tire_MFSwift/CPI Tire/Sensing Wheel Fixed Frame ==
  note: Incorrect - needs to be component
      | normal to ground plane
  Ang Velocity Vector : Subsystem
  Calculate Camber : Subsystem
  Dot Product : DotProduct  OutDataTypeStr=Inherit: Inherit via internal rule
  Dot Product1 : DotProduct  OutDataTypeStr=Inherit: Inherit via internal rule
  Dot Product2 : DotProduct  OutDataTypeStr=Inherit: Inherit via internal rule
  Get uvec Yaw axis : Subsystem
  PS-Simulink Converter1 : nesl_utility/PS-Simulink Converter  PhysicalDomain=network_engine_domain  SubClassName=ps_output  LeftPortType=input  RightPortType=output  PseudoPeriodic=off  Frequencies=[]  VectorFormat=1-D array  Unit=1  AffineConversion=off
  PS-Simulink Converter2 : nesl_utility/PS-Simulink Converter  PhysicalDomain=network_engine_domain  SubClassName=ps_output  LeftPortType=input  RightPortType=output  PseudoPeriodic=off  Frequencies=[]  VectorFormat=1-D array  Unit=1  AffineConversion=off
  PS-Simulink Converter6 : nesl_utility/PS-Simulink Converter  PhysicalDomain=network_engine_domain  SubClassName=ps_output  LeftPortType=input  RightPortType=output  PseudoPeriodic=off  Frequencies=[]  VectorFormat=1-D array  Unit=1  AffineConversion=off
  Project onto Road Plane : Subsystem
  Rot -90 deg about Z : Subsystem
  Select z axis : Selector  NumberOfDimensions=2  InputPortWidth=2  IndexOptions=Index vector (dialog),Index vector (dialog)  Indices=[1 2 3],3  OutputSizes=1,1
  Terminator : Terminator
  Transform Sensor Base : sm_lib/Frames and Transforms/Transform Sensor  MeasurementFrame=Base  RotationSequence=XYX  SenseAngle=off  SenseAxis=off  SenseQ=off  SenseR=on  SenseRotationSequence=off  SenseOmegaX=on  SenseOmegaY=on  SenseOmegaZ=on  SenseOmega=off  SenseQDot=off  SenseRDot=off  SenseRotationSequenceDot=off  SenseAlphaX=off  SenseAlphaY=off  SenseAlphaZ=off  SenseAlpha=off  SenseQDDot=off  SenseRDDot=off  SenseX=off  SenseY=off  SenseZ=on  SenseXYZ=off  SenseRad=off  SenseAzim=off  SenseDist=off  SenseInc=off  SenseXDot=on  SenseYDot=on  SenseZDot=on  SenseXYZDot=off  SenseRadDot=off  SenseAzimDot=off  SenseDistDot=off  SenseIncDot=off  SenseXDDot=off  SenseYDDot=off  SenseZDDot=off  SenseXYZDDot=off  SenseRadDDot=off  SenseAzimDDot=off  SenseDistDDot=off  SenseIncDDot=off
  Velocity Vector : Subsystem
  World Frame : sm_lib/Frames and Transforms/World Frame
  Whl : PMIOPort  Side=Left
  R : Outport  VectorParamsAs1DForOutWhenUnconnected=off
  vx : Outport  Port=2  VectorParamsAs1DForOutWhenUnconnected=off
  vy : Outport  Port=3  VectorParamsAs1DForOutWhenUnconnected=off
  Camber : Outport  Port=4  VectorParamsAs1DForOutWhenUnconnected=off
  yaw deriv : Outport  Port=5  VectorParamsAs1DForOutWhenUnconnected=off
  z : Outport  Port=6  VectorParamsAs1DForOutWhenUnconnected=off
  vz : Outport  Port=7  VectorParamsAs1DForOutWhenUnconnected=off
  wires:
  PS-Simulink Converter2/1 -> vz/1
  PS-Simulink Converter6/1 -> Select z axis/1, R/1
  Select z axis/1 -> Get uvec Yaw axis/1(zf), Calculate Camber/1(uvec spin axis), Project onto Road Plane/1(v), Terminator/1  "uvec spin axis"
  Rot -90 deg about Z/1(v rot -z) -> Dot Product1/2  "uvec whl long on ground"
  Velocity Vector/1(vxyz) -> Dot Product/2, Dot Product1/1  "vxyz Base"
  Get uvec Yaw axis/1(u) -> Dot Product2/2  "u"
  Ang Velocity Vector/1(wxyz) -> Dot Product2/1  "wxyz Base"
  Dot Product2/1 -> yaw deriv/1
  Project onto Road Plane/1(v proj) -> Rot -90 deg about Z/1(v), Dot Product/1  "uvec whl lat on ground"
  Dot Product/1 -> vy/1
  Dot Product1/1 -> vx/1
  PS-Simulink Converter1/1 -> z/1
  Calculate Camber/1(Camber) -> Camber/1
  connections:
  Transform Sensor Base/RConn1 -- Whl/RConn1
  PS-Simulink Converter6/LConn1 -- Transform Sensor Base/RConn2
  Transform Sensor Base/LConn1 -- World Frame/RConn1
  Transform Sensor Base/RConn3 -- Ang Velocity Vector/LConn1
  Ang Velocity Vector/LConn2 -- Transform Sensor Base/RConn4
  Transform Sensor Base/RConn5 -- Ang Velocity Vector/LConn3
  Velocity Vector/LConn1 -- Transform Sensor Base/RConn7
  Velocity Vector/LConn2 -- Transform Sensor Base/RConn8
  PS-Simulink Converter2/LConn1 -- Transform Sensor Base/RConn9 -- Velocity Vector/LConn3
  PS-Simulink Converter1/LConn1 -- Transform Sensor Base/RConn6
